simulink subsystem "att_det"  (R2022b)
settings: Solver=VariableStepAuto  StartTime=0.0  StopTime=10.0  RelTol=1e-3
settings Model: Creator=robertopistonenascone  LastModifiedBy=robertopistonenascone

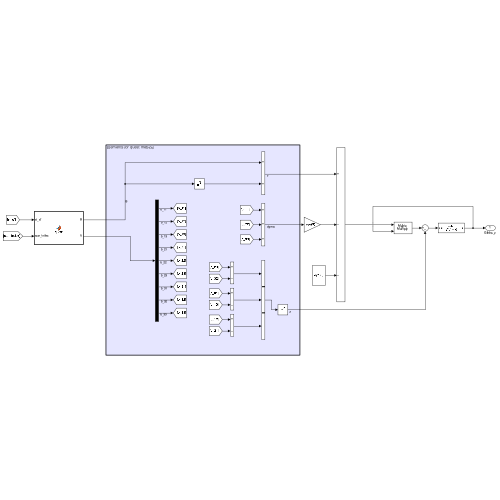
[thumbnail: Simulink's stored preview of the top-level diagram]
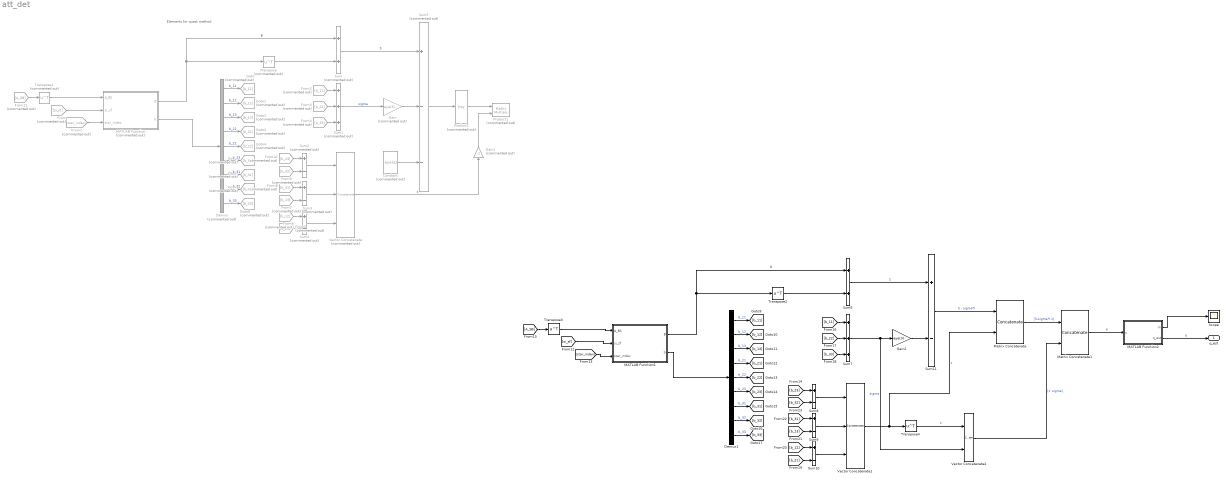
== system att_det ==
  note: Elements for quest method
  Constant : Constant  Commented=on  Value=eye(3)
  Demux : Demux  Commented=on  Outputs=9
  Demux1 : Demux  Outputs=9
  From : From  Commented=on  GotoTag=si_sf  TagVisibility=global
  From1 : From  Commented=on  GotoTag=star_index  TagVisibility=global
  From10 : From  Commented=on  GotoTag=b_23
  From11 : From  Commented=on  GotoTag=A_SB  TagVisibility=global
  From2 : From  Commented=on  GotoTag=b_11
  From3 : From  Commented=on  GotoTag=b_22
  From4 : From  Commented=on  GotoTag=b_33
  From5 : From  Commented=on  GotoTag=b_21
  From6 : From  Commented=on  GotoTag=b_12
  From7 : From  Commented=on  GotoTag=b_13
  From8 : From  Commented=on  GotoTag=b_31
  From9 : From  Commented=on  GotoTag=b_32
  Gain : Gain  Commented=on  Gain=eye(3)
  Gain1 : Gain  Commented=on  Gain=-1
  Gain2 : Gain  Gain=eye(3)
  Goto : Goto  Commented=on  GotoTag=b_11
  Goto1 : Goto  Commented=on  GotoTag=b_12
  Goto2 : Goto  Commented=on  GotoTag=b_13
  Goto3 : Goto  Commented=on  GotoTag=b_21
  Goto4 : Goto  Commented=on  GotoTag=b_22
  Goto5 : Goto  Commented=on  GotoTag=b_23
  Goto6 : Goto  Commented=on  GotoTag=b_31
  Goto7 : Goto  Commented=on  GotoTag=b_32
  Goto8 : Goto  Commented=on  GotoTag=b_33
  MATLAB Function : MATLAB Function  Commented=on  TreatAsAtomicUnit=on
  MATLAB Function1 : MATLAB Function  TreatAsAtomicUnit=on
  MATLAB Function2 : MATLAB Function  TreatAsAtomicUnit=on
  Matrix Concatenate : Concatenate  Mode=Multidimensional array  ConcatenateDimension=2
  Matrix Concatenate1 : Concatenate  Mode=Multidimensional array
  Product1 : Product  Commented=on  Multiplication=Matrix(*)
  Product2 : Product  Commented=on  Inputs=/  Multiplication=Matrix(*)  SaturateOnIntegerOverflow=on  OutDataTypeStr=Inherit: Same as first input
  Scope : Scope
  Sum : Sum  Commented=on
  Sum1 : Sum  Commented=on  Inputs=+++
  Sum{8..11} (4 alike) : Sum  Inputs=+-
  Sum2 : Sum  Commented=on  Inputs=+-
  Sum3 : Sum  Commented=on  Inputs=+-
  Sum4 : Sum  Commented=on  Inputs=+-
  Sum5 : Sum  Commented=on  Inputs=+--
  Sum6 : Sum
  Sum7 : Sum  Inputs=+++
  Transpose : Math  Commented=on  Operator=transpose
  Transpose1 : Math  Commented=on  Operator=transpose
  Transpose2 : Math  Operator=transpose
  Transpose3 : Math  Operator=transpose
  Transpose4 : Math  Operator=transpose
  Vector Concatenate : Concatenate  Commented=on  NumInputs=3  Mode=Multidimensional array
  Vector Concatenate1 : Concatenate  NumInputs=3  Mode=Multidimensional array
  Vector Concatenate2 : Concatenate
  q_est : Outport
  wires:
  MATLAB Function/1(B) -> Sum/1, Transpose/1  "B"
  From/1 -> MATLAB Function/2(si_sf)
  From1/1 -> MATLAB Function/3(star_index)
  Transpose/1 -> Sum/2
  Sum/1 -> Sum5/1  "S"
  MATLAB Function/2(b) -> Demux/1
  Sum1/1 -> Gain/1  "sigma"
  Demux/1 -> Goto/1  "b_11"
  Demux/2 -> Goto1/1  "b_12"
  Demux/3 -> Goto2/1  "b_13"
  Demux/4 -> Goto3/1  "b_21"
  Demux/5 -> Goto4/1  "b_22"
  Demux/6 -> Goto5/1  "b_23"
  Demux/7 -> Goto6/1  "b_31"
  Demux/8 -> Goto7/1  "b_32"
  Demux/9 -> Goto8/1  "b_33"
  From2/1 -> Sum1/1
  From3/1 -> Sum1/2
  From4/1 -> Sum1/3
  From10/1 -> Sum2/1
  From9/1 -> Sum2/2
  From8/1 -> Sum3/1
  From7/1 -> Sum3/2
  From6/1 -> Sum4/1
  From5/1 -> Sum4/2
  Sum3/1 -> Vector Concatenate/2
  Sum2/1 -> Vector Concatenate/1
  Sum4/1 -> Vector Concatenate/3
  Constant/1 -> Sum5/3
  Gain/1 -> Sum5/2
  Vector Concatenate/1 -> Gain1/1  "z"
  Gain1/1 -> Product1/2
  From11/1 -> Transpose1/1
  Transpose1/1 -> MATLAB Function/1(A_BS)
  Sum5/1 -> Product2/1
  Product2/1 -> Product1/1
  Sum7/1 -> Gain2/1, Vector Concatenate2/2  "sigma"
  MATLAB Function1/1(B) -> Sum6/1, Transpose2/1  "B"
  [b_31] -> Sum9/1
  Demux1/3 -> [b_13]  "b_13"
  Sum10/1 -> Vector Concatenate1/3
  Demux1/1 -> [b_11]  "b_11"
  [b_33] -> Sum7/3
  Demux1/6 -> [b_23]  "b_23"
  Demux1/5 -> [b_22]  "b_22"
  [b_12] -> Sum10/1
  [b_23] -> Sum8/1
  Demux1/4 -> [b_21]  "b_21"
  [b_11] -> Sum7/1
  MATLAB Function1/2(b) -> Demux1/1
  Transpose2/1 -> Sum6/2
  Sum6/1 -> Sum11/1  "S"
  [b_13] -> Sum9/2
  [b_21] -> Sum10/2
  [b_32] -> Sum8/2
  [b_22] -> Sum7/2
  Demux1/9 -> [b_33]  "b_33"
  Sum8/1 -> Vector Concatenate1/1
  Demux1/7 -> [b_31]  "b_31"
  Gain2/1 -> Sum11/2
  [star_index] -> MATLAB Function1/3(star_index)
  [si_sf] -> MATLAB Function1/2(si_sf)
  Demux1/8 -> [b_32]  "b_32"
  [A_SB] -> Transpose3/1
  Sum9/1 -> Vector Concatenate1/2
  Transpose3/1 -> MATLAB Function1/1(A_BS)
  Demux1/2 -> [b_12]  "b_12"
  Sum11/1 -> Matrix Concatenate/1  "S - sigma*I"
  Vector Concatenate1/1 -> Transpose4/1, Matrix Concatenate/2  "z"
  Transpose4/1 -> Vector Concatenate2/1  "z'"
  Vector Concatenate2/1 -> Matrix Concatenate1/2  "[z' sigma]"
  Matrix Concatenate/1 -> Matrix Concatenate1/1  "[S-sigma*I z]"
  Matrix Concatenate1/1 -> MATLAB Function2/1(u)  "K"
  MATLAB Function2/1(m) -> Scope/1
  MATLAB Function2/2(q_est) -> q_est/1  "q"

== matlab function att_det/MATLAB Function ==
  data: A_BS input; si_sf input; B output; star_index input; catalogue parameter; b output
function [B, b] = quest(A_BS, si_sf, star_index, catalogue)

B = zeros(3, 3);
vi = zeros(length(star_index), 3);


% vector of real star position
for k = 1:length(star_index)

    % check if the sensor is pointing correctly
    if star_index(k) == 0
        vi(k, :) = zeros(3,1);
    else
        vi(k, :) = catalogue(star_index(k), (1:3));
    end

    % rotation from sensor to body frame
    si_bf = A_BS*si_sf(k, :)';

    % create B matrix
    B = B + ( si_bf*vi(k, :) );

end
b = [B(1, 1) B(1, 2) B(1, 3) B(2, 1) B(2, 2) B(2, 3) B(3, 1) B(3, 2) B(3, 3)];

== matlab function att_det/MATLAB Function1 ==
  data: A_BS input; si_sf input; B output; star_index input; catalogue parameter; b output
function [B, b] = quest(A_BS, si_sf, star_index, catalogue)

B = zeros(3, 3);
vi = zeros(length(star_index), 3);


% vector of real star position
for k = 1:length(star_index)

    % check if the sensor is pointing correctly
    if star_index(k) == 0
        vi(k, :) = zeros(3,1);
    else
        vi(k, :) = catalogue(star_index(k), (1:3));
        vi(k, :) = vi(k, :)/(norm(vi(k, :)));
    end

    % rotation from sensor to body frame
    si_bf = A_BS*si_sf(k, :)';
    si_bf = si_bf/(norm(si_bf));

    % create B matrix
    B = B + ( si_bf*vi(k, :) );

end
b = [B(1, 1) B(1, 2) B(1, 3) B(2, 1) B(2, 2) B(2, 3) B(3, 1) B(3, 2) B(3, 3)];

== matlab function att_det/MATLAB Function2 ==
  data: m output; u input; q_est output
function [m, q_est] = fcn(u)

[q, lambda] = eig(u);
lambda_est = [lambda(1,1) lambda(2,2) lambda(3,3) lambda(4,4)];
[m, i] = max(real(lambda_est));
q_est = real(q(:, i));
